simulink model "matlab_loadflow_modified"  (R2014a)
settings: Solver=ode23t  StartTime=0.0  StopTime=1  RelTol=1e-3
libraries: powerlib x61
settings Model: Creator=Divya M  LastModifiedBy=Divya M
settings DebuggingCC: SolverPrmCheckMsg=none

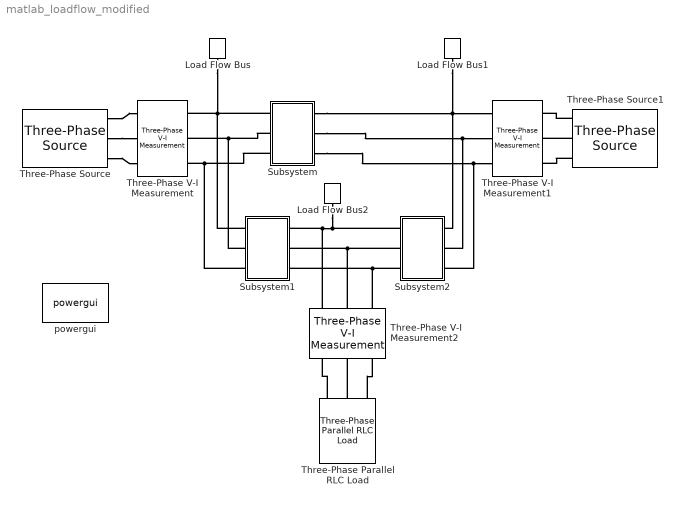
== system matlab_loadflow_modified ==
  Load Flow Bus : powerlib/Measurements/Load Flow Bus  LConnTagsString=a  ID=BUS_1  Vbase=230e3  Vref=1.05  Vangle=0  VLF=1  angleLF=0
      settings: AttributesFormatString=%<ID>\n%<Vbase>V\n%<VLF>pu\n%<angleLF>deg.
  Load Flow Bus1 : powerlib/Measurements/Load Flow Bus  LConnTagsString=a  ID=BUS_2  Vbase=230e3  Vref=1.07  Vangle=0  VLF=1  angleLF=0
      settings: AttributesFormatString=%<ID>\n%<Vbase>V\n%<VLF>pu\n%<angleLF>deg.
  Load Flow Bus2 : powerlib/Measurements/Load Flow Bus  LConnTagsString=a  ID=BUS_3  Vbase=230e3  Vref=1.05  Vangle=0  VLF=1  angleLF=0
      settings: AttributesFormatString=%<ID>\n%<Vbase>V\n%<VLF>pu\n%<angleLF>deg.
  Subsystem : Subsystem
  Subsystem1 : Subsystem
  Subsystem2 : Subsystem
  Three-Phase Parallel RLC Load : powerlib/Elements/Three-Phase Parallel RLC Load  LConnTagsString=A|B|C  Configuration=Y (grounded)  NominalVoltage=230e3  NominalFrequency=50  ActivePower=70e6  InductivePower=70e6  CapacitivePower=0  Measurements=None  LoadType=constant PQ
  Three-Phase V-I Measurement : powerlib/Measurements/Three-Phase V-I Measurement  VoltageMeasurement=no  SetLabelV=off  LabelV=Vabc  Vpu=off  VpuLL=off  CurrentMeasurement=no  SetLabelI=off  LabelI=Iabc  Ipu=off  Pbase=100e6  Vbase=500e3  OutputType=Complex  PhasorSimulation=off  PSBequivalent=0
  Three-Phase V-I Measurement1 : powerlib/Measurements/Three-Phase V-I Measurement  VoltageMeasurement=no  SetLabelV=off  LabelV=Vabc  Vpu=off  VpuLL=off  CurrentMeasurement=no  SetLabelI=off  LabelI=Iabc  Ipu=off  Pbase=100e6  Vbase=500e3  OutputType=Complex  PhasorSimulation=off  PSBequivalent=0
  Three-Phase V-I Measurement2 : powerlib/Measurements/Three-Phase V-I Measurement  VoltageMeasurement=no  SetLabelV=off  LabelV=Vabc  Vpu=off  VpuLL=off  CurrentMeasurement=no  SetLabelI=off  LabelI=Iabc  Ipu=off  Pbase=100e6  Vbase=500e3  OutputType=Complex  PhasorSimulation=off  PSBequivalent=0
  Three-Phase Source : powerlib/Electrical Sources/Three-Phase Source  Voltage=230e3  PhaseAngle=0  Frequency=50  InternalConnection=Yg  SpecifyImpedance=off  Resistance=0  Inductance=0  ShortCircuitLevel=100e6  BaseVoltage=230e3  XRratio=7  BusType=swing  Pref=0  Qref=0  Qmin=-inf  Qmax=inf
  Three-Phase Source1 : powerlib/Electrical Sources/Three-Phase Source  Voltage=230e3  PhaseAngle=0  Frequency=50  InternalConnection=Yg  SpecifyImpedance=off  Resistance=0  Inductance=0  ShortCircuitLevel=100e6  BaseVoltage=230e3  XRratio=7  BusType=PV  Pref=50e6  Qref=0  Qmin=-inf  Qmax=inf
  powergui : powerlib/powergui  Priority=1  SimulationMode=Continuous  SolverType=Tustin  SampleTime=50e-6  frequency=60  SPID=off  DisableSnubberDevices=off  DisableRonSwitches=off  DisableVfSwitches=off  SwTol=0  Interpol=off  DisplayEquations=off  Ts=0  methode=off  frequencyindice=50  Pbase=100e6  ErrMax=1e-4  Iterations=50  UnitsV=kV  UnitsW=MW  FunctionMessages=off  echomessages=off  HookPort=off  EnableUseOfTLC=off  x0status=blocks  RestoreLinks=warning  ResistiveCurrentMeasurement=off  Frange=[0:2:500]  Ylog=off  Xlog=on  ShowGrid=off  save=off  variable=ZData  structure=0  ZoomFFT=off  StartTime=0.0  cycles=1  DisplayStyle=1  fundamental=60  FreqAxis=off  MaxFrequency=1000  frequencyindicesteady=1  RmsSteady=1  display=off
  connections:
  Three-Phase Source/RConn1 -- Three-Phase V-I Measurement/LConn1
  Three-Phase Source/RConn2 -- Three-Phase V-I Measurement/LConn2
  Three-Phase Source/RConn3 -- Three-Phase V-I Measurement/LConn3
  Three-Phase Source1/RConn1 -- Three-Phase V-I Measurement1/LConn1
  Three-Phase Source1/RConn2 -- Three-Phase V-I Measurement1/LConn2
  Three-Phase Source1/RConn3 -- Three-Phase V-I Measurement1/LConn3
  Three-Phase Parallel RLC Load/LConn1 -- Three-Phase V-I Measurement2/LConn1
  Three-Phase Parallel RLC Load/LConn2 -- Three-Phase V-I Measurement2/LConn2
  Three-Phase Parallel RLC Load/LConn3 -- Three-Phase V-I Measurement2/LConn3
  Load Flow Bus1/LConn1 -- Subsystem2/RConn1 -- Subsystem/RConn1 -- Three-Phase V-I Measurement1/RConn1
  Load Flow Bus/LConn1 -- Subsystem1/LConn1 -- Subsystem/LConn1 -- Three-Phase V-I Measurement/RConn1
  Subsystem/LConn2 -- Subsystem1/LConn2 -- Three-Phase V-I Measurement/RConn2
  Subsystem/RConn2 -- Subsystem2/RConn2 -- Three-Phase V-I Measurement1/RConn2
  Subsystem/LConn3 -- Subsystem1/LConn3 -- Three-Phase V-I Measurement/RConn3
  Subsystem/RConn3 -- Subsystem2/RConn3 -- Three-Phase V-I Measurement1/RConn3
  Three-Phase V-I Measurement2/RConn1 -- Subsystem1/RConn1 -- Subsystem2/LConn1 -- Load Flow Bus2/LConn1
  Three-Phase V-I Measurement2/RConn2 -- Subsystem2/LConn2 -- Subsystem1/RConn2
  Three-Phase V-I Measurement2/RConn3 -- Subsystem2/LConn3 -- Subsystem1/RConn3

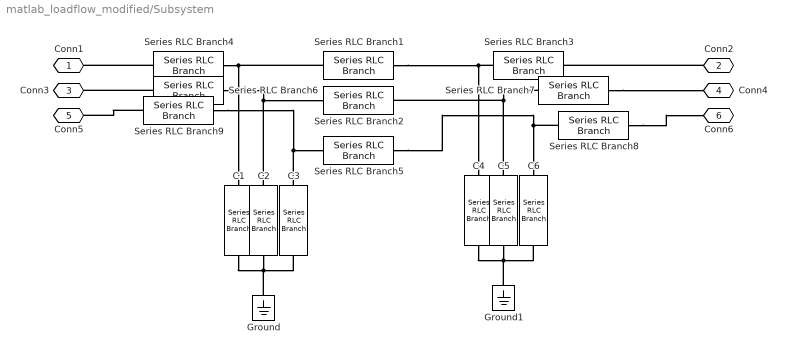
== system matlab_loadflow_modified/Subsystem ==
  C{1..6} (6 alike) : powerlib/Elements/Series RLC Branch  LConnTagsString=__new0  RConnTagsString=__new0  BranchType=C  Resistance=1  Inductance=1e-3  SetiL0=off  InitialCurrent=0  Capacitance=0.01*2/314  Setx0=off  InitialVoltage=0  Measurements=None
  Ground : powerlib/Elements/Ground  LConnTagsString=a
  Ground1 : powerlib/Elements/Ground  LConnTagsString=a
  Series RLC Branch1 : powerlib/Elements/Series RLC Branch  LConnTagsString=__new0  RConnTagsString=__new0  BranchType=RL  Resistance=0.1  Inductance=0.2/314  SetiL0=off  InitialCurrent=0  Capacitance=1e-6  Setx0=off  InitialVoltage=0  Measurements=None
  Series RLC Branch2 : powerlib/Elements/Series RLC Branch  LConnTagsString=__new0  RConnTagsString=__new0  BranchType=RL  Resistance=0.1  Inductance=0.2/314  SetiL0=off  InitialCurrent=0  Capacitance=1e-6  Setx0=off  InitialVoltage=0  Measurements=None
  Series RLC Branch{3..4,6..9} (6 alike) : powerlib/Elements/Series RLC Branch  LConnTagsString=__new0  RConnTagsString=__new0  BranchType=R  Resistance=0.000001  Inductance=0.2/314  SetiL0=off  InitialCurrent=0  Capacitance=1e-6  Setx0=off  InitialVoltage=0  Measurements=None
  Series RLC Branch5 : powerlib/Elements/Series RLC Branch  LConnTagsString=__new0  RConnTagsString=__new0  BranchType=RL  Resistance=0.1  Inductance=0.2/314  SetiL0=off  InitialCurrent=0  Capacitance=1e-6  Setx0=off  InitialVoltage=0  Measurements=None
  Conn1 : PMIOPort  Port=1  Side=Left
  Conn2 : PMIOPort  Port=2  Side=Right
  Conn3 : PMIOPort  Port=3  Side=Left
  Conn4 : PMIOPort  Port=4  Side=Right
  Conn5 : PMIOPort  Port=5  Side=Left
  Conn6 : PMIOPort  Port=6  Side=Right
  connections:
  C5/LConn1 -- Series RLC Branch7/LConn1 -- Series RLC Branch2/RConn1
  Series RLC Branch1/LConn1 -- Series RLC Branch4/RConn1 -- C1/LConn1
  C2/LConn1 -- Series RLC Branch6/RConn1 -- Series RLC Branch2/LConn1
  C3/LConn1 -- Series RLC Branch9/RConn1 -- Series RLC Branch5/LConn1
  Series RLC Branch1/RConn1 -- Series RLC Branch3/LConn1 -- C4/LConn1
  Series RLC Branch5/RConn1 -- Series RLC Branch8/LConn1 -- C6/LConn1
  C1/RConn1 -- C3/RConn1 -- Ground/LConn1 -- C2/RConn1
  C4/RConn1 -- C5/RConn1 -- Ground1/LConn1 -- C6/RConn1
  Conn2/RConn1 -- Series RLC Branch3/RConn1
  Series RLC Branch4/LConn1 -- Conn1/RConn1
  Series RLC Branch6/LConn1 -- Conn3/RConn1
  Series RLC Branch9/LConn1 -- Conn5/RConn1
  Series RLC Branch7/RConn1 -- Conn4/RConn1
  Series RLC Branch8/RConn1 -- Conn6/RConn1

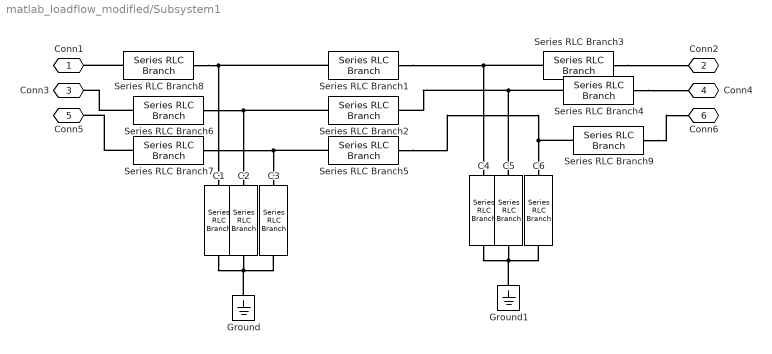
== system matlab_loadflow_modified/Subsystem1 ==
  C{1..6} (6 alike) : powerlib/Elements/Series RLC Branch  LConnTagsString=__new0  RConnTagsString=__new0  BranchType=C  Resistance=1  Inductance=1e-3  SetiL0=off  InitialCurrent=0  Capacitance=0.01*2/314  Setx0=off  InitialVoltage=0  Measurements=None
  Ground : powerlib/Elements/Ground  LConnTagsString=a
  Ground1 : powerlib/Elements/Ground  LConnTagsString=a
  Series RLC Branch1 : powerlib/Elements/Series RLC Branch  LConnTagsString=__new0  RConnTagsString=__new0  BranchType=RL  Resistance=0.05  Inductance=0.2/314  SetiL0=off  InitialCurrent=0  Capacitance=1e-6  Setx0=off  InitialVoltage=0  Measurements=None
  Series RLC Branch2 : powerlib/Elements/Series RLC Branch  LConnTagsString=__new0  RConnTagsString=__new0  BranchType=RL  Resistance=0.05  Inductance=0.2/314  SetiL0=off  InitialCurrent=0  Capacitance=1e-6  Setx0=off  InitialVoltage=0  Measurements=None
  Series RLC Branch{3..4,6..9} (6 alike) : powerlib/Elements/Series RLC Branch  LConnTagsString=__new0  RConnTagsString=__new0  BranchType=R  Resistance=0.000001  Inductance=0.2/314  SetiL0=off  InitialCurrent=0  Capacitance=1e-6  Setx0=off  InitialVoltage=0  Measurements=None
  Series RLC Branch5 : powerlib/Elements/Series RLC Branch  LConnTagsString=__new0  RConnTagsString=__new0  BranchType=RL  Resistance=0.05  Inductance=0.2/314  SetiL0=off  InitialCurrent=0  Capacitance=1e-6  Setx0=off  InitialVoltage=0  Measurements=None
  Conn1 : PMIOPort  Port=1  Side=Left
  Conn2 : PMIOPort  Port=2  Side=Right
  Conn3 : PMIOPort  Port=3  Side=Left
  Conn4 : PMIOPort  Port=4  Side=Right
  Conn5 : PMIOPort  Port=5  Side=Left
  Conn6 : PMIOPort  Port=6  Side=Right
  connections:
  C5/RConn1 -- C4/RConn1 -- C6/RConn1 -- Ground1/LConn1
  C2/RConn1 -- Ground/LConn1 -- C3/RConn1 -- C1/RConn1
  Series RLC Branch5/RConn1 -- Series RLC Branch9/LConn1 -- C6/LConn1
  Series RLC Branch1/RConn1 -- Series RLC Branch3/LConn1 -- C4/LConn1
  Series RLC Branch5/LConn1 -- Series RLC Branch7/RConn1 -- C3/LConn1
  Series RLC Branch2/LConn1 -- Series RLC Branch6/RConn1 -- C2/LConn1
  Series RLC Branch1/LConn1 -- Series RLC Branch8/RConn1 -- C1/LConn1
  C5/LConn1 -- Series RLC Branch2/RConn1 -- Series RLC Branch4/LConn1
  Series RLC Branch8/LConn1 -- Conn1/RConn1
  Series RLC Branch3/RConn1 -- Conn2/RConn1
  Series RLC Branch4/RConn1 -- Conn4/RConn1
  Series RLC Branch6/LConn1 -- Conn3/RConn1
  Series RLC Branch7/LConn1 -- Conn5/RConn1
  Series RLC Branch9/RConn1 -- Conn6/RConn1

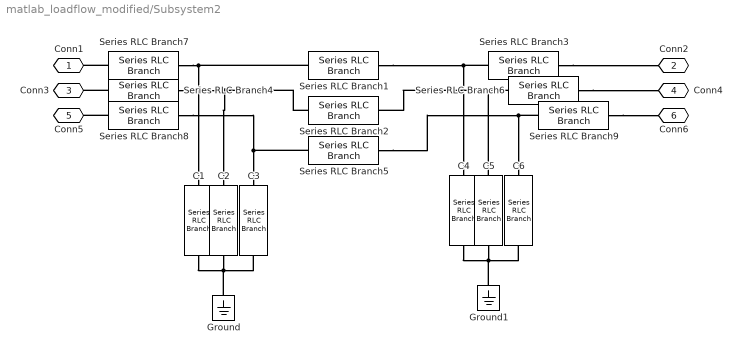
== system matlab_loadflow_modified/Subsystem2 ==
  C{1..6} (6 alike) : powerlib/Elements/Series RLC Branch  LConnTagsString=__new0  RConnTagsString=__new0  BranchType=C  Resistance=1  Inductance=1e-3  SetiL0=off  InitialCurrent=0  Capacitance=0.03/314  Setx0=off  InitialVoltage=0  Measurements=None
  Ground : powerlib/Elements/Ground  LConnTagsString=a
  Ground1 : powerlib/Elements/Ground  LConnTagsString=a
  Series RLC Branch1 : powerlib/Elements/Series RLC Branch  LConnTagsString=__new0  RConnTagsString=__new0  BranchType=RL  Resistance=0.08  Inductance=0.3/314  SetiL0=off  InitialCurrent=0  Capacitance=1e-6  Setx0=off  InitialVoltage=0  Measurements=None
  Series RLC Branch2 : powerlib/Elements/Series RLC Branch  LConnTagsString=__new0  RConnTagsString=__new0  BranchType=RL  Resistance=0.08  Inductance=0.3/314  SetiL0=off  InitialCurrent=0  Capacitance=1e-6  Setx0=off  InitialVoltage=0  Measurements=None
  Series RLC Branch{3..4,6..9} (6 alike) : powerlib/Elements/Series RLC Branch  LConnTagsString=__new0  RConnTagsString=__new0  BranchType=R  Resistance=0.000001  Inductance=0.2/314  SetiL0=off  InitialCurrent=0  Capacitance=1e-6  Setx0=off  InitialVoltage=0  Measurements=None
  Series RLC Branch5 : powerlib/Elements/Series RLC Branch  LConnTagsString=__new0  RConnTagsString=__new0  BranchType=RL  Resistance=0.08  Inductance=0.3/314  SetiL0=off  InitialCurrent=0  Capacitance=1e-6  Setx0=off  InitialVoltage=0  Measurements=None
  Conn1 : PMIOPort  Port=1  Side=Left
  Conn2 : PMIOPort  Port=2  Side=Right
  Conn3 : PMIOPort  Port=3  Side=Left
  Conn4 : PMIOPort  Port=4  Side=Right
  Conn5 : PMIOPort  Port=5  Side=Left
  Conn6 : PMIOPort  Port=6  Side=Right
  connections:
  C5/RConn1 -- C4/RConn1 -- C6/RConn1 -- Ground1/LConn1
  C2/RConn1 -- Ground/LConn1 -- C3/RConn1 -- C1/RConn1
  Series RLC Branch5/RConn1 -- Series RLC Branch9/LConn1 -- C6/LConn1
  Series RLC Branch1/RConn1 -- Series RLC Branch3/LConn1 -- C4/LConn1
  Series RLC Branch5/LConn1 -- C3/LConn1 -- Series RLC Branch8/RConn1
  Series RLC Branch2/LConn1 -- C2/LConn1 -- Series RLC Branch4/RConn1
  Series RLC Branch1/LConn1 -- Series RLC Branch7/RConn1 -- C1/LConn1
  C5/LConn1 -- Series RLC Branch6/LConn1 -- Series RLC Branch2/RConn1
  Series RLC Branch7/LConn1 -- Conn1/RConn1
  Series RLC Branch3/RConn1 -- Conn2/RConn1
  Series RLC Branch4/LConn1 -- Conn3/RConn1
  Series RLC Branch6/RConn1 -- Conn4/RConn1
  Series RLC Branch8/LConn1 -- Conn5/RConn1
  Series RLC Branch9/RConn1 -- Conn6/RConn1
